simulink subsystem "ControlLeds"  (R2024b)
settings: Solver=VariableStepAuto  StartTime=0.0  StopTime=10.0  RelTol=1e-3
libraries: simulink x4
settings Model: Creator=Laura  LastModifiedBy=Laura

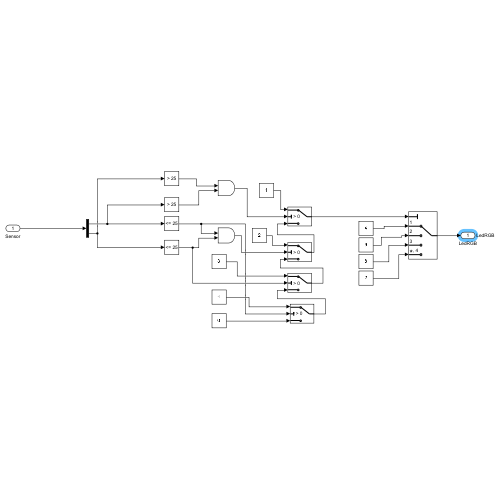
[thumbnail: Simulink's stored preview of the top-level diagram]
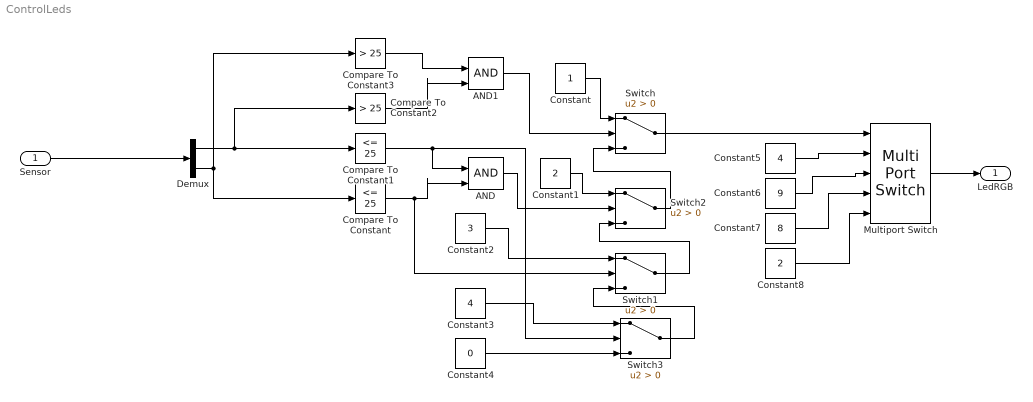
== system ControlLeds ==
  Sensor : Inport
  AND : Logic  IconShape=distinctive  AllPortsSameDT=off  OutDataTypeStr=boolean
  AND1 : Logic  IconShape=distinctive  AllPortsSameDT=off  OutDataTypeStr=boolean
  Compare To Constant : simulink/Logic and Bit Operations/Compare To Constant  relop=<=  const=25  OutDataTypeStr=boolean
  Compare To Constant1 : simulink/Logic and Bit Operations/Compare To Constant  relop=<=  const=25  OutDataTypeStr=boolean
  Compare To Constant2 : simulink/Logic and Bit Operations/Compare To Constant  relop=>  const=25  OutDataTypeStr=boolean
  Compare To Constant3 : simulink/Logic and Bit Operations/Compare To Constant  relop=>  const=25  OutDataTypeStr=boolean
  Constant : Constant
  Constant1 : Constant  Value=2
  Constant2 : Constant  Value=3
  Constant3 : Constant  Value=4
  Constant4 : Constant  Value=0
  Constant5 : Constant  Value=4
  Constant6 : Constant  Value=9
  Constant7 : Constant  Value=8
  Constant8 : Constant  Value=2
  Demux : Demux  Outputs=2
  Multiport Switch : MultiPortSwitch  Inputs=4  SaturateOnIntegerOverflow=off  InputSameDT=off
  Switch{,1..3} (4 alike) : Switch  Criteria=u2 > Threshold  SaturateOnIntegerOverflow=off  InputSameDT=off
  LedRGB : Outport  SignalName=LedRGB
  wires:
  Sensor/1 -> Demux/1
  Demux/1 -> Compare To Constant2/1, Compare To Constant1/1
  Demux/2 -> Compare To Constant/1, Compare To Constant3/1
  Compare To Constant/1 -> Switch1/2, AND/2
  Compare To Constant1/1 -> Switch3/2, AND/1
  Compare To Constant3/1 -> AND1/1
  Compare To Constant2/1 -> AND1/2
  AND1/1 -> Switch/2
  Constant/1 -> Switch/1
  Switch/1 -> Multiport Switch/1
  Switch2/1 -> Switch/3
  AND/1 -> Switch2/2
  Constant1/1 -> Switch2/1
  Switch1/1 -> Switch2/3
  Constant2/1 -> Switch1/1
  Switch3/1 -> Switch1/3
  Constant3/1 -> Switch3/1
  Constant4/1 -> Switch3/3
  Constant5/1 -> Multiport Switch/2
  Constant6/1 -> Multiport Switch/3
  Constant7/1 -> Multiport Switch/4
  Constant8/1 -> Multiport Switch/5
  Multiport Switch/1 -> LedRGB/1
